simulink model "PV1000_STM32_767_ZI_state_control"  (R2023a)
settings: Solver=FixedStepAuto  StartTime=0.0  StopTime=inf  FixedStep=0.001  RelTol=1e-3
undefined symbols (not defined in the file): DiscIntNeverNeededParam
libraries: mbedblockslib x17, simulink x14, slpidlib x3, stmnucleolib x2, nucleoutilitieslib x1, etargetslib x1, dspswit3 x1
(part 2 of 2)

== matlab function PV1000_STM32_767_ZI_state_control/AMS6915, I2C Bus 2/AMS6915_calculate pressure2 ==
  data: digoutp input; p output
% Function performs conversion from digital output of the sensor to
% physical units
%%%%%%%%%%%%%%%%%%%%%%%%%%%%%%%%%%%%%%%%%%%%%%%%%%%%%%%%%%%%%%%%%%%%%%%%%
% Input arguments: 
% digoutp - 14-bit value containig the H- & L_Byte of the pressure value 
% Output arguments:
% p - Pressure in mbar
%%%%%%%%%%%%%%%%%%%%%%%%%%%%%%%%%%%%%%%%%%%%%%%%%%%%%%%%%%%%%%%%%%%%%%%%%

function p = AMS6915_calculate_pressure(digoutp)
% Unpack the data bits
digoutp_HB = digoutp(1,1); % High Byte (last 6 (low) bits are data bits)
digoutp_LB = digoutp(2,1); % Low Byte  (all bits are data bits)
temp_byte = hex2dec('3F');
% Calculate the measured T_raw and convert it to double
p_raw =  single(bitand(digoutp_HB,temp_byte))*256  + single(digoutp_LB);
% Scaling formula
p = ((p_raw - 1638)/(13107/200)) - 100;

== matlab function PV1000_STM32_767_ZI_state_control/AMS 6915, I2C Bus 4/AMS6915_calculate pressure3 ==
  data: digoutp input; p output
% Function performs conversion from digital output of the sensor to
% physical units
%%%%%%%%%%%%%%%%%%%%%%%%%%%%%%%%%%%%%%%%%%%%%%%%%%%%%%%%%%%%%%%%%%%%%%%%%
% Input arguments: 
% digoutp - 14-bit value containig the H- & L_Byte of the pressure value 
% Output arguments:
% p - Pressure in mbar
%%%%%%%%%%%%%%%%%%%%%%%%%%%%%%%%%%%%%%%%%%%%%%%%%%%%%%%%%%%%%%%%%%%%%%%%%

function p = AMS6915_calculate_pressure(digoutp)
% Unpack the data bits
digoutp_HB = digoutp(1,1); % High Byte (last 6 (low) bits are data bits)
digoutp_LB = digoutp(2,1); % Low Byte  (all bits are data bits)
temp_byte = hex2dec('3F');
% Calculate the measured T_raw and convert it to double
p_raw =  single(bitand(digoutp_HB,temp_byte))*256  + single(digoutp_LB);
% Scaling formula
p = ((p_raw - 1638)/(13107/200)) - 100;

== matlab function PV1000_STM32_767_ZI_state_control/AMS 6915, I2C Bus 4/AMS6915_calculate_temperature3 ==
  data: digoutT input; T output
% Function performs conversion from digital output of the sensor to
% physical units
%%%%%%%%%%%%%%%%%%%%%%%%%%%%%%%%%%%%%%%%%%%%%%%%%%%%%%%%%%%%%%%%%%%%%%%%%
% Input arguments: 
% digoutT - 12-bit value containig the H- & L_Byte of the temperature value 
% Output arguments:
% T - Temperature in Degree Celsius
%%%%%%%%%%%%%%%%%%%%%%%%%%%%%%%%%%%%%%%%%%%%%%%%%%%%%%%%%%%%%%%%%%%%%%%%%


function T = AMS6915_calculate_Temperature(digoutT)


% Unpack the input vectors
digoutT_HB = digoutT(3,1); % High byte (all bits are data bits)
digoutT_LB = digoutT(4,1); % Low byte  (first 3 (high) bits are data bits)
temp_byte = hex2dec('07');
% Calculate the measured T_raw and convert to double
T_raw = single(digoutT_HB)*8 + single(bitand(bitsrl(digoutT_LB,5),temp_byte));
% Scaling formula
T = ((T_raw*200)/2048) - 50;

== matlab function PV1000_STM32_767_ZI_state_control/SFM3300, I2C Bus 4/Enabled Subsystem5/MATLAB Function ==
  data: digoutQ_insp input; Q_insp output
% Function performs conversion from digital output of the sensor to
% physical units
%%%%%%%%%%%%%%%%%%%%%%%%%%%%%%%%%%%%%%%%%%%%%%%%%%%%%%%%%%%%%%%%%%%%%%%%%
% Input arguments: 
% digoutQ_insp - 16-bit value containig the H- & L_Byte of the flow value 
% Output arguments:
% Q_insp - Flow in slm
%%%%%%%%%%%%%%%%%%%%%%%%%%%%%%%%%%%%%%%%%%%%%%%%%%%%%%%%%%%%%%%%%%%%%%%%%

function Q_insp = SFM3300_calculate_insp_flow(digoutQ_insp)
% Unpack the data bits
digoutQ_insp_HB = digoutQ_insp(1,1); % High Byte (all bits are data bits)
digoutQ_insp_LB = digoutQ_insp(2,1); % Low Byte  (all bits are data bits)
% Calculate the measured Q_insp_raw and convert to double
Q_insp_raw =  single(digoutQ_insp_HB)*256  + single(digoutQ_insp_LB);
% Scaling formula
Q_insp = (Q_insp_raw - 32768)/120 ;

== matlab function PV1000_STM32_767_ZI_state_control/SFM3300, I2C Bus 4/MATLAB Function2 ==
  data: digoutQ_insp input; Q_insp output
% Function performs conversion from digital output of the sensor to
% physical units
%%%%%%%%%%%%%%%%%%%%%%%%%%%%%%%%%%%%%%%%%%%%%%%%%%%%%%%%%%%%%%%%%%%%%%%%%
% Input arguments: 
% digoutQ_insp - 16-bit value containig the H- & L_Byte of the flow value 
% Output arguments:
% Q_insp - Flow in slm
%%%%%%%%%%%%%%%%%%%%%%%%%%%%%%%%%%%%%%%%%%%%%%%%%%%%%%%%%%%%%%%%%%%%%%%%%

function Q_insp = SFM3300_calculate_insp_flow(digoutQ_insp)
% Unpack the data bits
digoutQ_insp_HB = digoutQ_insp(1,1); % High Byte (all bits are data bits)
digoutQ_insp_LB = digoutQ_insp(2,1); % Low Byte  (all bits are data bits)
% Calculate the measured Q_insp_raw and convert to double
Q_insp_raw =  single(digoutQ_insp_HB)*256  + single(digoutQ_insp_LB);
% Scaling formula
Q_insp = (Q_insp_raw - 32768)/120.0 ;

== matlab function PV1000_STM32_767_ZI_state_control/AMS6915, I2C Bus 2/AMS6915_calculate_temperature2 ==
  data: digoutT input; T output
% Function performs conversion from digital output of the sensor to
% physical units
%%%%%%%%%%%%%%%%%%%%%%%%%%%%%%%%%%%%%%%%%%%%%%%%%%%%%%%%%%%%%%%%%%%%%%%%%
% Input arguments: 
% digoutT - 12-bit value containig the H- & L_Byte of the temperature value 
% Output arguments:
% T - Temperature in Degree Celsius
%%%%%%%%%%%%%%%%%%%%%%%%%%%%%%%%%%%%%%%%%%%%%%%%%%%%%%%%%%%%%%%%%%%%%%%%%


function T = AMS6915_calculate_Temperature(digoutT)


% Unpack the input vectors
digoutT_HB = digoutT(3,1); % High byte (all bits are data bits)
digoutT_LB = digoutT(4,1); % Low byte  (first 3 (high) bits are data bits)
temp_byte = hex2dec('07');
% Calculate the measured T_raw and convert to double
T_raw = single(digoutT_HB)*8 + single(bitand(bitsrl(digoutT_LB,5),temp_byte));
% Scaling formula
T = ((T_raw*200)/2048) - 50;

== stateflow chart PV1000_STM32_767_ZI_state_control/State_and_Reference_Trajectory/MainControl ==
  settings: sampleTime=1e-3  executeAtInitialization=1
  state Standby/
    entry:
    isMandInsp = false;
    isInspPause = false;
    isPControlled = false;
    isStandby = true;
    exit:
    isStandby = false;
  state PressureMandatoryVentilation/ %PCV ; no trigger at the moment
    entry:
    state MVExp/
      entry:
      isMandInsp = false;
    state MVInsp/
      entry:
      isMandInsp = true;
      isPControlled = true;
    (default) -> MVExp
    MVInsp -> MVExp : after(TimeInsp,sec)
    MVExp -> MVInsp : after(TimeExp, sec)
  state FlowMandatoryVentilation/ % VCV ; no trigger at the moment
    entry:
    state VCVInsp/
      state FlowInsp/
        entry:
        isMandInsp = true;
        isPControlled = false;
      state FlowInspPause
        entry:
        isMandInsp = true;
        isInspPause = true;
      (default) -> FlowInsp
      FlowInsp -> FlowInspPause [order 2] : [enPMAX]
      FlowInsp -> FlowInspPause [order 1] : after(TimeInsp - TimeInspPause, sec)
    state FlowExp/
      entry:
      isMandInsp = false;
      isInspPause = false;
    VCVInsp -> FlowExp : after(TimeInsp, sec)
    (default) -> FlowExp
    FlowExp -> VCVInsp : after(TimeExp, sec)
  (default) -> ? [order 1]
  (default) -> Standby [order 1]
  (junction 630) -> Standby [order 1] : [Mode==4]
  Standby -> (junction 630) : [Mode!=4]
  (junction 630) -> PressureMandatoryVentilation/ %PCV ; no trigger at the moment [order 2] : [Mode==2]
  (junction 639) -> (junction 630)
  (junction 630) -> FlowMandatoryVentilation/ % VCV ; no trigger at the moment [order 3] : [Mode==3]
  PressureMandatoryVentilation/ %PCV ; no trigger at the moment -> (junction 639) : [Mode!=2]
  (junction 625) -> (junction 639)
  FlowMandatoryVentilation/ % VCV ; no trigger at the moment -> (junction 625) : [Mode!=3]
  data: VExp_m local double; isPControlled output boolean; isMandInsp output boolean; Mode input single; TimeInsp input single; TimeInspPause input single; TimeExp input single; VTidal_set input single; isInspPause output boolean; allOff output boolean; isStandby output boolean; enPMAX input boolean

== stateflow chart PV1000_STM32_767_ZI_state_control/State_and_Reference_Trajectory/Boundary Check/Chart ==
  settings: executeAtInitialization=1
  state spcv/
    entry:
    mode = 2;
  state standby/
    entry:
    mode = 4;
  state svcv/
    entry:
    mode = 3;
  (default) -> standby
  standby -> spcv [order 1] : [mode_in == 2]
  spcv -> standby [order 2] : [mode_in ~= 2]
  svcv -> standby [order 2] : [mode_in ~= 3]
  standby -> svcv [order 2] : [mode_in == 3]
  spcv -> svcv [order 1] : [mode_in == 3]
  svcv -> spcv [order 1] : [mode_in == 2]
  data: data local single; mode output single; mode_in input single
  events: change_mode input EITHER_EDGE_EVENT

== stateflow chart PV1000_STM32_767_ZI_state_control/State_and_Reference_Trajectory/TrajectoryPlanning ==
  settings: sampleTime=0.01
  state Standby/
    entry:
    PInsp_ref = 0;
    FInsp_ref = 0;
    PEEP_ref = 0;
    O2_ref = 0;
  state Ventilation
    state MandInspP/
      entry:
      PInsp_ref = PInsp_set;
      FInsp_ref = 0;
      PEEP_ref = PEEP_set;
      O2_ref = O2_set;
      exit:
      PInsp_ref = PEEP_set;
    state MandInspF/
      entry:
      PInsp_ref = PMax_set;
      FInsp_ref = VTidal_set / (TimeInsp_set-TimeInspPause_set) * 0.06;
      PEEP_ref = PEEP_set;
      O2_ref = O2_set;
      exit:
      PInsp_ref = PEEP_set;
      FInsp_ref = 0;
    state exp/
      entry:
      PInsp_ref = PEEP_set;
      O2_ref = O2_set;
    state MandInspFInspPause/
      exit:
      PInsp_ref = PEEP_set;
      FInsp_ref = 0;
    (default) -> (junction 89) : {PInsp_ref = PEEP_set;
        | PEEP_ref = PEEP_set;}
    MandInspP -> (junction 73) : [ !isMandInsp]
    (junction 73) -> (junction 74)
    (junction 89) -> MandInspP [order 1] : [isMandInsp && isPControlled]
    exp -> (junction 89) : [isMandInsp ]
    (junction 89) -> (junction 79) [order 2]
    (junction 79) -> MandInspF [order 1] : [isMandInsp && !isPControlled]
    (junction 79) -> (junction 82) [order 2]
    MandInspF -> (junction 74) [order 2] : [!isMandInsp]
    MandInspF -> MandInspFInspPause [order 1] : [isInspPause]
    (junction 107) -> exp
    MandInspFInspPause -> (junction 74) : [!isMandInsp]
    (junction 74) -> (junction 82)
    (junction 82) -> (junction 107)
  (default) -> Standby
  Ventilation -> Standby : [isStandby]
  Standby -> Ventilation : [!isStandby]
  data: isStandby input boolean; isPControlled input boolean size=1; isMandInsp input boolean size=1; isInspPause input boolean; PInsp_set input single size=1; PMax_set input single; PEEP_set input single size=1; VTidal_set input single; O2_set input single size=1; TimeInsp_set input single; TimeInspPause_set input single; PInsp_ref output single size=1; PEEP_ref output single size=1; FInsp_ref output single size=1; O2_ref output single size=1

== matlab function PV1000_STM32_767_ZI_state_control/SFM3019, I2C Bus 4/MATLAB Function3 ==
  data: digoutQ_exp input; Q_exp output
% Function performs conversion from digital output of the sensor to
% physical units
%%%%%%%%%%%%%%%%%%%%%%%%%%%%%%%%%%%%%%%%%%%%%%%%%%%%%%%%%%%%%%%%%%%%%%%%%
% Input arguments: 
% digoutQ_exp - 16-bit value containig the H- & L_Byte of the flow value 
% Output arguments:
% Q_exp - Flow in slm
%%%%%%%%%%%%%%%%%%%%%%%%%%%%%%%%%%%%%%%%%%%%%%%%%%%%%%%%%%%%%%%%%%%%%%%%%

function Q_exp = SFM3019_calculate_insp_flow(digoutQ_exp)
% Unpack the data bits
digoutQ_exp_HB = digoutQ_exp(1,1); % High Byte (int) (all bits are data bits)
digoutQ_exp_LB = digoutQ_exp(2,1); % Low Byte (int)  (all bits are data bits)
% Calculate the measured Q_exp_raw and convert to double
Q_exp_raw =  single(digoutQ_exp_HB)*256  + single(digoutQ_exp_LB);
% Scaling formula
Q_exp = (Q_exp_raw + 24576)/170.0 ;

== matlab function PV1000_STM32_767_ZI_state_control/SFM3300, I2C Bus 2/Enabled Subsystem1/MATLAB Function ==
  data: digoutQ_insp input; Q_insp output
% Function performs conversion from digital output of the sensor to
% physical units
%%%%%%%%%%%%%%%%%%%%%%%%%%%%%%%%%%%%%%%%%%%%%%%%%%%%%%%%%%%%%%%%%%%%%%%%%
% Input arguments: 
% digoutQ_insp - 16-bit value containig the H- & L_Byte of the flow value 
% Output arguments:
% Q_insp - Flow in slm
%%%%%%%%%%%%%%%%%%%%%%%%%%%%%%%%%%%%%%%%%%%%%%%%%%%%%%%%%%%%%%%%%%%%%%%%%

function Q_insp = SFM3300_calculate_insp_flow(digoutQ_insp)
% Unpack the data bits
digoutQ_insp_HB = digoutQ_insp(1,1); % High Byte (all bits are data bits)
digoutQ_insp_LB = digoutQ_insp(2,1); % Low Byte  (all bits are data bits)
% Calculate the measured Q_insp_raw and convert to double
Q_insp_raw =  single(digoutQ_insp_HB)*256  + single(digoutQ_insp_LB);
% Scaling formula
Q_insp = (Q_insp_raw - 32768)/120 ;

== matlab function PV1000_STM32_767_ZI_state_control/SFM3300, I2C Bus 2/MATLAB Function1 ==
  data: digoutQ_insp input; Q_insp output
% Function performs conversion from digital output of the sensor to
% physical units
%%%%%%%%%%%%%%%%%%%%%%%%%%%%%%%%%%%%%%%%%%%%%%%%%%%%%%%%%%%%%%%%%%%%%%%%%
% Input arguments: 
% digoutQ_insp - 16-bit value containig the H- & L_Byte of the flow value 
% Output arguments:
% Q_insp - Flow in slm
%%%%%%%%%%%%%%%%%%%%%%%%%%%%%%%%%%%%%%%%%%%%%%%%%%%%%%%%%%%%%%%%%%%%%%%%%

function Q_insp = SFM3300_calculate_insp_flow(digoutQ_insp)
% Unpack the data bits
digoutQ_insp_HB = digoutQ_insp(1,1); % High Byte (all bits are data bits)
digoutQ_insp_LB = digoutQ_insp(2,1); % Low Byte  (all bits are data bits)
% Calculate the measured Q_insp_raw and convert to double
Q_insp_raw =  single(digoutQ_insp_HB)*256  + single(digoutQ_insp_LB);
% Scaling formula
Q_insp = (Q_insp_raw - 32768)/120.0 ;
